simulink model "prac_p1"  (R2024a)
settings: Solver=VariableStepAuto  StartTime=0.0  StopTime=2500  RelTol=1e-3
libraries: simulink x1
settings Model: Creator=heman  LastModifiedBy=heman

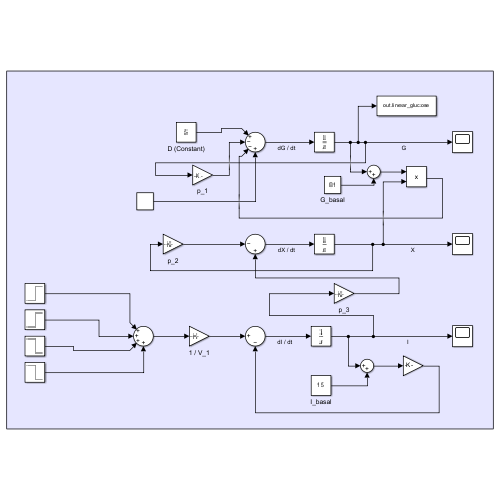
[thumbnail: Simulink's stored preview of the top-level diagram]
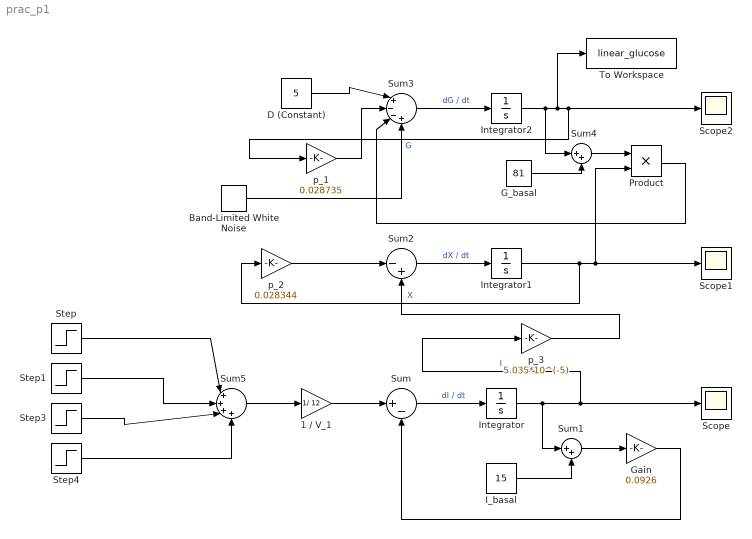
== system prac_p1 ==
  1 / V_1 : Gain  Gain=1/ 12
  Band-Limited White Noise : simulink/Sources/Band-Limited White Noise  Cov=[0.1]  Ts=0.1  seed=[23341]
  D (Constant) : Constant  Value=5
  G_basal : Constant  Value=81
  Gain : Gain  Gain=0.0926
  I_basal : Constant  Value=15
  Integrator : Integrator
  Integrator1 : Integrator
  Integrator2 : Integrator
  Product : Product
  Scope : Scope
  Scope1 : Scope
  Scope2 : Scope
  Step : Step  Time=500  Before=25  After=27.5  SampleTime=0
  Step1 : Step  Time=1000  After=2.5  SampleTime=0
  Step3 : Step  Time=1500  After=-2.5  SampleTime=0
  Step4 : Step  Time=2000  After=-2.5  SampleTime=0
  Sum : Sum  Inputs=|+-
  Sum1 : Sum  Inputs=|++
  Sum2 : Sum  Inputs=|-+
  Sum3 : Sum  Inputs=|+--+
  Sum4 : Sum  Inputs=|++
  Sum5 : Sum  Inputs=|++++
  To Workspace : ToWorkspace  VariableName=linear_glucose  SampleTime=-1
  p_1 : Gain  Gain=0.028735
  p_2 : Gain  Gain=0.028344
  p_3 : Gain  Gain=5.035*10^(-5)
  wires:
  Sum5/1 -> 1 / V_1/1
  1 / V_1/1 -> Sum/1
  Sum/1 -> Integrator/1  "dI / dt"
  Integrator/1 -> Sum1/1, p_3/1, Scope/1  "I"
  I_basal/1 -> Sum1/2
  Sum1/1 -> Gain/1
  Gain/1 -> Sum/2
  Sum2/1 -> Integrator1/1  "dX / dt"
  Integrator1/1 -> p_2/1, Product/2, Scope1/1  "X"
  p_3/1 -> Sum2/2
  p_2/1 -> Sum2/1
  Sum3/1 -> Integrator2/1  "dG / dt"
  Integrator2/1 -> Sum4/1, To Workspace/1, p_1/1, Scope2/1  "G"
  G_basal/1 -> Sum4/2
  Sum4/1 -> Product/1
  D (Constant)/1 -> Sum3/1
  p_1/1 -> Sum3/2
  Product/1 -> Sum3/3
  Step/1 -> Sum5/1
  Step1/1 -> Sum5/2
  Step3/1 -> Sum5/3
  Step4/1 -> Sum5/4
  Band-Limited White Noise/1 -> Sum3/4
